simulink model "MidSnap"  (R2020a)
settings: configuration reference "testConfig" (kept outside this file)
model workspace (MAT data in the model file):
  midSnapParam = Simulink.Parameter
  midSnapParam.Value = 3
  midSnapParam.DataType = 'int32'
  midSnapParam.Dimensions = [1 1]
settings Model: DataDictionary=TestConfig.sldd  ParameterArgumentNames=midSnapParam  OrderedModelArguments=off  Creator=raarenst  LastModifiedBy=toma
settings ConfigSetRef: SourceName=testConfig

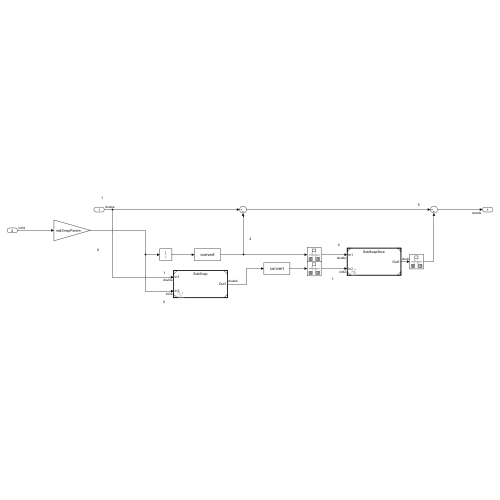
[thumbnail: Simulink's stored preview of the top-level diagram]
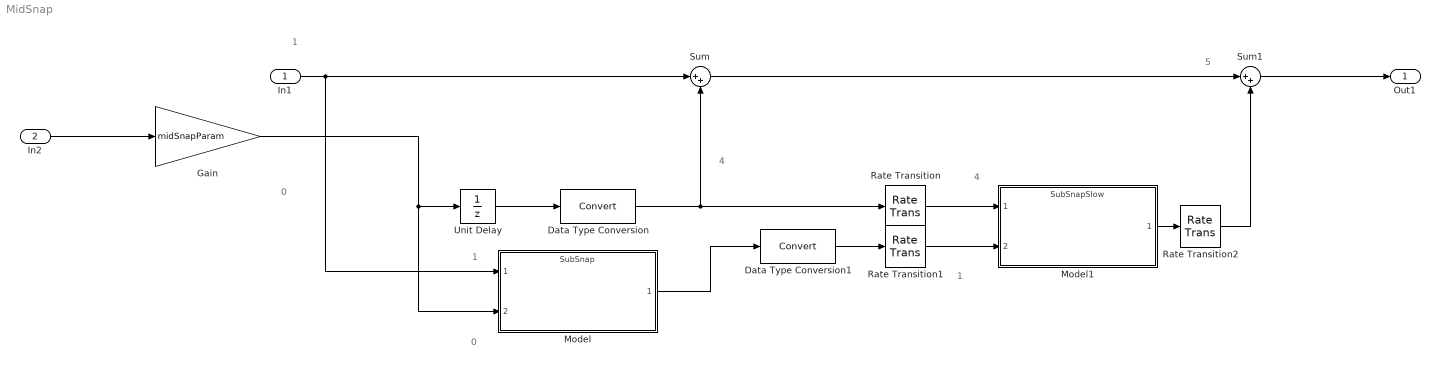
== system MidSnap ==
  note: 1
  note: 5
  note: 4
  note: 0
  note: 1
  note: 0
  note: 1
  note: 4
  In1 : Inport  OutDataTypeStr=double  SampleTime=0.1
  In2 : Inport  Port=2  OutDataTypeStr=int32  SampleTime=0.1
  Data Type Conversion : DataTypeConversion
  Data Type Conversion1 : DataTypeConversion
  Gain : Gain  Gain=midSnapParam  OutDataTypeStr=int32
  Model : ModelReference  ModelNameDialog=SubSnap  SimulationMode=Normal  ModelReferenceVersion=1.1
  Model1 : ModelReference  ModelNameDialog=SubSnapSlow  SimulationMode=Normal  ModelReferenceVersion=1.1
  Rate Transition : RateTransition
  Rate Transition1 : RateTransition
  Rate Transition2 : RateTransition
  Sum : Sum  Inputs=|++
  Sum1 : Sum  Inputs=|++
  Unit Delay : UnitDelay  InitialCondition=4  SampleTime=-1  HasFrameUpgradeWarning=on
  Out1 : Outport  OutDataTypeStr=double
  wires:
  In2/1 -> Gain/1
  Gain/1 -> Unit Delay/1, Model/2
  Unit Delay/1 -> Data Type Conversion/1
  In1/1 -> Sum/1, Model/1
  Data Type Conversion/1 -> Rate Transition/1, Sum/2
  Sum/1 -> Sum1/1
  Model/1 -> Data Type Conversion1/1
  Sum1/1 -> Out1/1
  Model1/1 -> Rate Transition2/1
  Data Type Conversion1/1 -> Rate Transition1/1
  Rate Transition/1 -> Model1/1
  Rate Transition1/1 -> Model1/2
  Rate Transition2/1 -> Sum1/2
